simulink subsystem "robot"  (R2021b)
settings: Solver=VariableStepAuto  StartTime=0.0  StopTime=10.0  RelTol=1e-3
settings Model: Creator=marco  LastModifiedBy=marco

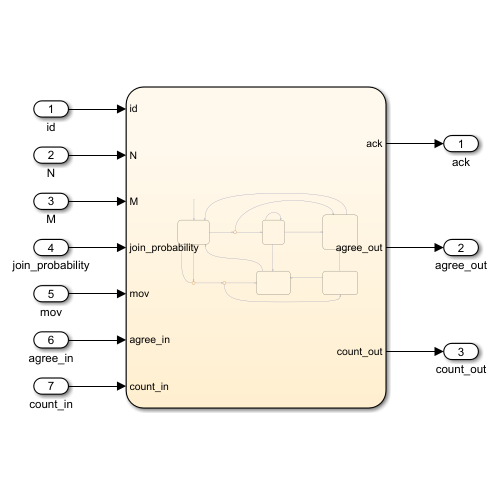
[thumbnail: Simulink's stored preview of the top-level diagram]
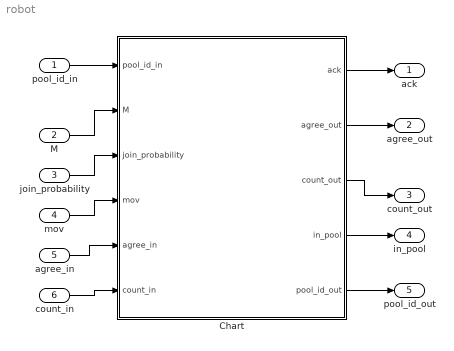
== system robot ==
  pool_id_in : Inport
  M : Inport  Port=2
  join_probability : Inport  Port=3
  mov : Inport  Port=4
  agree_in : Inport  Port=5
  count_in : Inport  Port=6
  Chart : Stateflow chart  TreatAsAtomicUnit=on
  ack : Outport
  agree_out : Outport  Port=2
  count_out : Outport  Port=3
  in_pool : Outport  Port=4
  pool_id_out : Outport  Port=5
  wires:
  pool_id_in/1 -> Chart/1(pool_id_in)
  M/1 -> Chart/2(M)
  join_probability/1 -> Chart/3(join_probability)
  Chart/1(ack) -> ack/1
  Chart/2(agree_out) -> agree_out/1
  Chart/3(count_out) -> count_out/1
  mov/1 -> Chart/4(mov)
  agree_in/1 -> Chart/5(agree_in)
  count_in/1 -> Chart/6(count_in)
  Chart/4(in_pool) -> in_pool/1
  Chart/5(pool_id_out) -> pool_id_out/1

== stateflow chart robot/Chart ==
  state Abort
    entry:
    if (~is_coord)
    agree_out = -1;
    else
    ack = -1;
    end
    exit:
    agree_out = 0;
    ack = 0;
  state MovWait
    entry:
    is_coord = 0;
    pool_id_out = 0;
    during:
    count_out = 0;
    agree_out = agree_in;
  state Coordination
    during:
    count_out = 0;
    agree_out = 0;
  state CommonAction
    entry:
    in_pool = 1;
    during:
    agree_out = 0;
    ack = 0;
    % count_out = count_in;
    exit:
    in_pool = 0;
  state AgreeWait
    entry:
    count_out = count_in + 1;
    during:
    count_out = 0;
  Abort -> MovWait
  (junction 99) -> Abort [order 2]
  (default) -> MovWait : {join = (join_probability > 0.5);}
  Coordination -> Coordination [order 1] : % pool failed
      | [count_in > 0]
      | {agree_out = -1;}
  Coordination -> Abort [order 3] : % failure
      | [agree_in == -1]
  MovWait -> (junction 99) [order 1] : % request received
      | [mov]
      | {is_coord = 1;
      | pool_id_out = pool_id_in;}
  (junction 99) -> Coordination [order 1] : [join]
      | {count_out = 1;}
  Coordination -> CommonAction [order 2] : % success
      | [agree_in == 1]
      | {ack = 1;}
  (junction 105) -> MovWait [order 2] : {count_out = count_in;}
  MovWait -> (junction 105) [order 2] : % query to commit
      | [count_in > 0]
  CommonAction -> MovWait : after(2,sec)
  AgreeWait -> Abort [order 2] : % failure
      | [agree_in == -1]
  (junction 105) -> (junction 111) [order 1] : [join]
      | {pool_id_out = pool_id_in;}
  (junction 111) -> CommonAction [order 1] : % pool formed
      | [count_in+1 == M]
      | {agree_out = 1;}
  (junction 111) -> AgreeWait [order 2] : % agree
  AgreeWait -> CommonAction [order 1] : % commit
      | [agree_in == 1]
      | {agree_out = 1;}
  data: pool_id_in input; M input; join_probability input; join local; mov input; ack output =0; agree_in input; count_in input; agree_out output =0; count_out output =0; is_coord local =0; in_pool output =0; pool_id_out output
